simulink model "visualservo7"  (R2014a)
settings: Solver=ode45  StartTime=0.0  StopTime=10.0  RelTol=1e-3
undefined symbols (not defined in the file): gray, IsPositionTracked, IsSkeletonTracked, JointDepthIndices, JointImageIndices, JointTrackingState, JointWorldCoordinates, none, PositionDepthIndices, PositionImageIndices, PositionWorldCoordinates, SegmentationData, SkeletonTrackingID, videoinput
libraries: simulink x7, fl_lib x7, elec_lib x4, nesl_utility x4, visionstatistics x1, visiontextngfix x1, imaqlib x1, vs x1, dspstat3 x1, dspindex x1, visionsinks x1
settings Model: Creator=lenovo  LastModifiedBy=lenovo

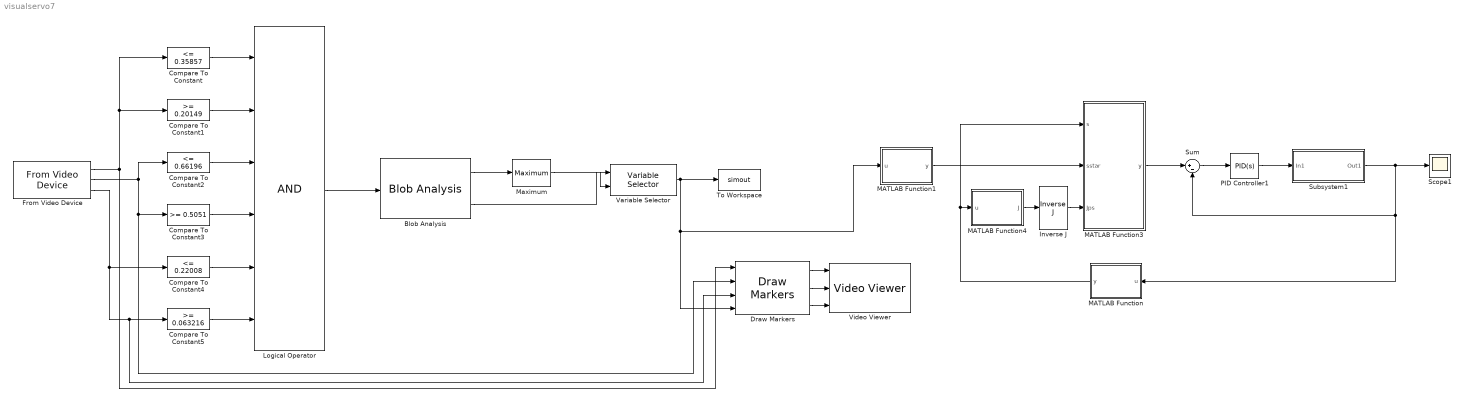
== system visualservo7 ==
  Blob Analysis : visionstatistics/Blob Analysis  Tag=vipblks_row_conv  area=on  centroid=on  bBox=off  majorAxis=off  minorAxis=off  angle=off  eccentricity=off  equivDiameterSq=off  extent=off  perimeter=off  maxBlobs=50  warnIfNumBlobsExceeded=on  isCount=off  useMinArea=off  minArea=0  useMaxArea=off  maxArea=intmax('uint32')  excludeBorderBlob=off  outDT=double  isOutVarDim=off  isFill=on  fillValues=-1  conn=8  isLabel=off  outputMode=Binary point scaling  outputWordLength=32  outputFracLength=16  firstCoeffMode=Binary point scaling  firstCoeffWordLength=16  firstCoeffFracLength=14  secondCoeffMode=Binary point scaling  secondCoeffWordLength=32  secondCoeffFracLength=16  accumMode=Binary point scaling  accumWordLength=32  accumFracLength=0  prodOutputMode=Binary point scaling  prodOutputWordLength=32  prodOutputFracLength=16  roundingMode=Floor  overflowMode=off
  Compare To Constant : simulink/Logic and Bit Operations/Compare To Constant  relop=<=  const=0.35857  OutDataTypeStr=boolean
  Compare To Constant1 : simulink/Logic and Bit Operations/Compare To Constant  relop=>=  const=0.20149  OutDataTypeStr=boolean
  Compare To Constant2 : simulink/Logic and Bit Operations/Compare To Constant  relop=<=  const=0.66196  OutDataTypeStr=boolean
  Compare To Constant3 : simulink/Logic and Bit Operations/Compare To Constant  relop=>=  const=0.5051  OutDataTypeStr=boolean
  Compare To Constant4 : simulink/Logic and Bit Operations/Compare To Constant  relop=<=  const=0.22008  OutDataTypeStr=boolean
  Compare To Constant5 : simulink/Logic and Bit Operations/Compare To Constant  relop=>=  const=0.063216  OutDataTypeStr=boolean
  Draw Markers : visiontextngfix/Draw Markers  shape=Square  size=3  fill=off  fillClrSource=Specify via dialog  display=White  intensity=200  color=[200 255 100]  opacity=0.6  viewport=Entire image  antialiasing=off  inType=Obsolete  imagePorts=Separate color signals  prodOutputMode=Binary point scaling  prodOutputWordLength=32  prodOutputFracLength=14  memoryMode=Specify word length  memoryWordLength=16  memoryFracLength=15  roundingMode=Floor  overflowMode=off
  From Video Device : imaqlib/From Video Device  DeviceMenu=winvideo 1 (Lenovo EasyCamera)  Device=winvideo 1 (Lenovo EasyCamera)  ObjConstructor=videoinput('winvideo', 1)  VideoFormatMenu=YUY2_800x600  VideoFormat=YUY2_800x600  VideoSource=input1  ROIPosition=[0 0 600 800]  EnableHWTrigger=off  TriggerConfiguration=none/none  SampleTime=1/30  OutputPortsMode=Separate color signals  DataType=single  CanDoHWTrigger=no  ReturnedColorSpace=rgb  BlockHandle=4022.0007  ROIWidth=800  ROIHeight=600  ROIColumn=0  ROIRow=0  EngXMLPath=C:\Program Files\MATLAB\R2014a\toolbox\imaq\imaq\private  DevXMLPath=C:\MATLAB\SupportPackages\R2014a\genericvideo\adaptor\win64  EngLibPath=C:\Program Files\MATLAB\R2014a\toolbox\imaq\imaqblks\imaqmex\win64  ColorSpace=rgb  BayerSensorAlignment=grbg  AllMetadata=IsPositionTracked;IsSkeletonTracked;JointDepthIndices;JointImageIndices;JointTrackingState;JointWorldCoordinates;PositionDepthIndices;PositionImageIndices;PositionWorldCoordinates;SegmentationData;SkeletonTrackingID
  Inverse J : vs/Jacobian/Inverse J
  Logical Operator : Logic  Inputs=6  AllPortsSameDT=off  OutDataTypeStr=boolean
  MATLAB Function : MATLAB Function  TreatAsAtomicUnit=on
  MATLAB Function1 : MATLAB Function  TreatAsAtomicUnit=on
  MATLAB Function3 : MATLAB Function  TreatAsAtomicUnit=on
  MATLAB Function4 : MATLAB Function  TreatAsAtomicUnit=on
  Maximum : dspstat3/Maximum  fcn=Value  reset=None  InputProcessing=Columns as channels (frame based)  indexBase=One  operateOver=Each column  Dimension=1  colComp=on  operation=maximum  roiEnable=off  roiType=Rectangles  roiPortion=Entire ROI  roiOutput=Individual statistics for each ROI  roiFlag=off  accumDataTypeStr=Inherit: Same as product output  accumLastDataTypeStr=Inherit: Same as product output  roundingMode=Floor  overflowMode=off
  PID Controller1 : simulink/Continuous/PID Controller  Controller=PID  TimeDomain=Continuous-time  SampleTime=1  IntegratorMethod=Forward Euler  FilterMethod=Forward Euler  Form=Parallel  P=0.000170731517770763  I=0.000499641743355433  D=1.72516596313632e-06  N=115.572730511561  InitialConditionSource=internal  InitialConditionForIntegrator=0  InitialConditionForFilter=0  ExternalReset=none  LimitOutput=off  UpperSaturationLimit=inf  LowerSaturationLimit=-inf  LinearizeAsGain=on  AntiWindupMode=none  Kb=1  TrackingMode=off  Kt=1  PParamMin=[]  PParamMax=[]  IParamMin=[]  IParamMax=[]  DParamMin=[]  DParamMax=[]  NParamMin=[]  NParamMax=[]  KbParamMin=[]  KbParamMax=[]  KtParamMin=[]  KtParamMax=[]  POutMin=[]  POutMax=[]  IOutMin=[]  IOutMax=[]  DOutMin=[]  DOutMax=[]  NOutMin=[]  NOutMax=[]  KbOutMin=[]  KbOutMax=[]  KtOutMin=[]  KtOutMax=[]  IntegratorOutMin=[]  IntegratorOutMax=[]  FilterOutMin=[]  FilterOutMax=[]  SumOutMin=[]  SumOutMax=[]  SumI1OutMin=[]  SumI1OutMax=[]  SumI2OutMin=[]  SumI2OutMax=[]  SumI3OutMin=[]  SumI3OutMax=[]  SumDOutMin=[]  SumDOutMax=[]  SaturationOutMin=[]  SaturationOutMax=[]  IntegratorContinuousStateAttributes=''  IntegratorStateMustResolveToSignalObject=off  IntegratorRTWStateStorageClass=Auto  FilterContinuousStateAttributes=''  FilterStateMustResolveToSignalObject=off  FilterRTWStateStorageClass=Auto
  Scope1 : Scope
      settings: YMin=3.2  SaveName=ScopeData2
  Subsystem1 : Subsystem
  Sum : Sum  Inputs=|+-
  To Workspace : ToWorkspace  VariableName=simout  SaveFormat=Timeseries  SampleTime=-1
  Variable Selector : dspindex/Variable Selector  NumInputs=1  rowsOrCols=Rows  IdxMode=Variable  Elements=[1 3]  ZerOneIdxMode=One-based  errmode=Clip Index  FillMode=on  FillValues=0
  Video Viewer : visionsinks/Video Viewer  inputType=Obsolete7b  imagePorts=Separate color signals  useColorMap=off  colormapValue=gray(256)  specRange=off  minInputVal=0  maxInputVal=255  FigPos=[707 685 517 290]  AxisZoom=on  trueSizedOnce=off  OpenAtMdlStart=on  DefaultConfigurationName=vipscopes.VideoViewerScopeCfg
  wires:
  Compare To Constant/1 -> Logical Operator/1
  Compare To Constant1/1 -> Logical Operator/2
  Compare To Constant2/1 -> Logical Operator/3
  Compare To Constant3/1 -> Logical Operator/4
  Compare To Constant4/1 -> Logical Operator/5
  Compare To Constant5/1 -> Logical Operator/6
  Logical Operator/1 -> Blob Analysis/1
  Blob Analysis/1 -> Maximum/1
  Variable Selector/1 -> Draw Markers/4, MATLAB Function1/1(u), To Workspace/1
  Maximum/1 -> Variable Selector/2
  Blob Analysis/2 -> Variable Selector/1
  From Video Device/1 -> Draw Markers/1, Compare To Constant/1, Compare To Constant1/1
  From Video Device/2 -> Compare To Constant2/1, Compare To Constant3/1, Draw Markers/2
  From Video Device/3 -> Draw Markers/3, Compare To Constant5/1, Compare To Constant4/1
  Draw Markers/1 -> Video Viewer/1
  Draw Markers/2 -> Video Viewer/2
  Draw Markers/3 -> Video Viewer/3
  Subsystem1/1(Out1) -> Scope1/1, MATLAB Function/1(u), Sum/2
  PID Controller1/1 -> Subsystem1/1(In1)
  Sum/1 -> PID Controller1/1
  MATLAB Function3/1(y) -> Sum/1
  MATLAB Function/1(y) -> MATLAB Function4/1(u), MATLAB Function3/1(s)
  Inverse J/1 -> MATLAB Function3/3(Jps)
  MATLAB Function1/1(y) -> MATLAB Function3/2(sstar)
  MATLAB Function4/1(J) -> Inverse J/1

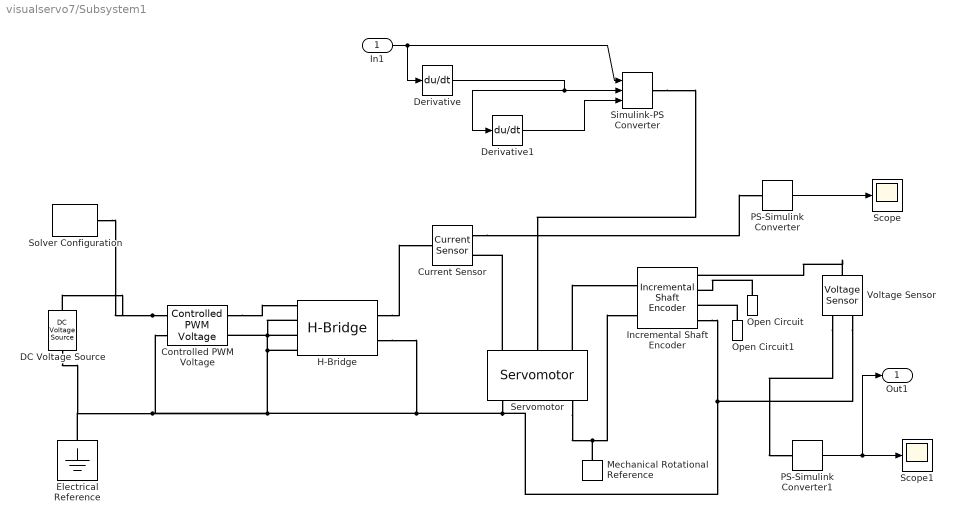
== system visualservo7/Subsystem1 ==
  In1 : Inport
  Controlled PWM Voltage : elec_lib/Actuators & Drivers/Drivers/Controlled PWM Voltage  F=1000 Hz  TD=0 s  pulse_width_offset=0 s  Vmin=0 V  Vmax=12 V  Vm=12 V  pwm_or_av=1  event_type=1  sample_time=1e-6 s
  Current Sensor : fl_lib/Electrical/Electrical Sensors/Current Sensor
  DC Voltage Source : fl_lib/Electrical/Electrical Sources/DC Voltage Source  v0=12 V
  Derivative : Derivative
  Derivative1 : Derivative
  Electrical Reference : fl_lib/Electrical/Electrical Elements/Electrical Reference
  H-Bridge : elec_lib/Actuators & Drivers/Drivers/H-Bridge  Venable=2.5 V  Vmax=5.0 V  Vreverse=2.5 V  Vbrake=2.5 V  Vm=12 V  pwm_or_av=1  discontinuous=0  freewheeling_mode=1  freewheeling_mode_disc=1  Ron=0.1 Ohm  Don=0.05 Ohm  Rload=10 Ohm  Lload=1e-5 H  F=10 kHz  w_vec=[1, 2] s  i_vec=[1, 2] A  vMatrix=[1, 2; 3, 4] V
  Incremental Shaft Encoder : elec_lib/Sensors/Incremental Shaft Encoder  NPulse=120  Vm=5 V  angle0=0 deg
  Mechanical Rotational Reference : fl_lib/Mechanical/Rotational Elements/Mechanical Rotational Reference
  Open Circuit : fl_lib/Electrical/Electrical Elements/Open Circuit
  Open Circuit1 : fl_lib/Electrical/Electrical Elements/Open Circuit
  PS-Simulink Converter : nesl_utility/PS-Simulink Converter  PhysicalDomain=network_engine_domain  SubClassName=ps_output  LeftPortType=input  RightPortType=output  PseudoPeriodic=off  Frequencies=[]  Unit=1  AffineConversion=off
  PS-Simulink Converter1 : nesl_utility/PS-Simulink Converter  PhysicalDomain=network_engine_domain  SubClassName=ps_output  LeftPortType=input  RightPortType=output  PseudoPeriodic=off  Frequencies=[]  Unit=1  AffineConversion=off
  Scope : Scope
      settings: YMin=0
  Scope1 : Scope
      settings: YMin=3.2
  Servomotor : elec_lib/Actuators & Drivers/Rotational Actuators/Servomotor  torque_speed_param=1  w_t=[ 0 3.75e+3 7.5e+3 8e+3 ] rpm  T_t=[0.09 0.08 0.07 0] N*m  torque_max=0.1 N*m  power_max=30 W  Tc=0.02 s  eff=100  w_eff=3.75e+3 rpm  T_eff=0.08 N*m  Piron=0 W  Pbase=0 W  Res=0 Ohm  J=5e-6 kg*m^2  lam=1e-5 N*m/(rad/s)  speed0=0 rpm  alpha=0.00393 1/K  Tmeas=25 C  thermal_mass=100 J/K  initial_temperature=25 C
  Simulink-PS Converter : nesl_utility/Simulink-PS Converter  PhysicalDomain=network_engine_domain  SubClassName=ps_input  LeftPortType=input  RightPortType=output  PseudoPeriodic=off  Frequencies=[]  NoiseDistribution=none  NoiseParameters=[]  Unit=1  AffineConversion=off  InputFiltering=derivs  SimscapeFilterOrder=1  InputFilterTimeConstant=0.001  UdotUserProvided=2
  Solver Configuration : nesl_utility/Solver Configuration  PhysicalDomain=network_engine_domain  SubClassName=solver  LeftPortType=input  RightPortType=generic  Accelerate=off  Tones=[]  Harmonics=[]  SimulateNoise=off  Profile=off  UseLocalSampling=off  EnableSwitchedLinearOptims=on  FrequencyDomain=off  UseCCode=off  RelTol=0.001  AbsTol=1e-06  MinStep=1e-09  ToWorkspace=off  DoDC=off  ResidualTolerance=1e-09  UseLocalSolver=off  LocalSolverChoice=NE_BACKWARD_EULER_ADVANCER  LocalSolverSampleTime=0.001  DoFixedCost=off  MaxNonlinIter=3  MaxModeIter=2  LinearAlgebra=Sparse  DelaysMemoryBudget=1024  AutomaticFiltering=on  FilteringTimeConstant=0.001
  Voltage Sensor : fl_lib/Electrical/Electrical Sensors/Voltage Sensor
  Out1 : Outport
  wires:
  PS-Simulink Converter/1 -> Scope/1
  PS-Simulink Converter1/1 -> Out1/1, Scope1/1
  In1/1 -> Simulink-PS Converter/1, Derivative/1
  Derivative/1 -> Derivative1/1, Simulink-PS Converter/2
  Derivative1/1 -> Simulink-PS Converter/3
  connections:
  Controlled PWM Voltage/LConn1 -- Solver Configuration/RConn1 -- DC Voltage Source/LConn1
  Incremental Shaft Encoder/RConn4 -- Controlled PWM Voltage/LConn2 -- Electrical Reference/LConn1 -- DC Voltage Source/RConn1 -- Controlled PWM Voltage/RConn2 -- H-Bridge/LConn2 -- H-Bridge/LConn3 -- H-Bridge/LConn4 -- H-Bridge/RConn2 -- Servomotor/RConn1 -- Voltage Sensor/RConn2
  Servomotor/RConn3 -- Mechanical Rotational Reference/LConn1 -- Incremental Shaft Encoder/LConn2
  Current Sensor/RConn1 -- PS-Simulink Converter/LConn1
  Simulink-PS Converter/RConn1 -- Servomotor/LConn2
  H-Bridge/RConn1 -- Current Sensor/LConn1
  Servomotor/LConn1 -- Current Sensor/RConn2
  Controlled PWM Voltage/RConn1 -- H-Bridge/LConn1
  Servomotor/LConn3 -- Incremental Shaft Encoder/LConn1
  Voltage Sensor/LConn1 -- Incremental Shaft Encoder/RConn1
  Voltage Sensor/RConn1 -- PS-Simulink Converter1/LConn1
  Open Circuit/LConn1 -- Incremental Shaft Encoder/RConn2
  Open Circuit1/LConn1 -- Incremental Shaft Encoder/RConn3

== matlab function visualservo7/MATLAB Function1 ==
  data: u input; y output
function y = fcn(u)
%#codegen

y = u(1:2)

== matlab function visualservo7/MATLAB Function ==
  data: u input; y output
function y = fcn(u)
%#codegen

y = [0;u];

== matlab function visualservo7/MATLAB Function3 ==
  data: s input; y output; sstar input; Jps input
function y = fcn(s,sstar,Jps)
%#codegen
Vc=Jps*(s-transpose(sstar));
y=Vc(1,1);

== matlab function visualservo7/MATLAB Function4 ==
  data: u input; J output
function J = fcn(u)
%#codegen
J=[-1 0 0 0 -1 u(2);0 -1 u(2) 1+(u(2))^2 0 0];
